simulink model "Detailed_Simulation_recogface_finger_yolo"  (R2023b)
settings: Solver=VariableStepAuto  StartTime=0.0  StopTime=100000  RelTol=1e-3
StartFcn:
  | %url_dc = 'http://localhost:51310/aas/joint_mechanism_1_aas/submodels/joint_mechanism_specific_submodel/elements/DampingCoefficient';
  | %response = webread(url_dc);
  | %set_param('Detailed_Simulation_v15_aas_if_V192_168_179_2/Revolute Joint1/','DampingCoefficient', response.elem.value);
  | %url_lal = 'http://localhost:51310/aas/joint_mechanism_1_aas/submodels/joint_mechanism_specific_submodel/elements/LowerAngleLimit';
  | %response = webread(url_lal);
  | 
  | %set_param('Detailed_Simulation_v15_aas_if_V192_168_179_2/Revolute Joint1/','LowerLimitBound','-45');
undefined symbols (not defined in the file): f, X, Y, Z
libraries: sm_lib x22, nesl_utility x7, slrealtimeutilitieslib x3, instrumentlib x2, slrealtimeiplib x1, dspnetwork x1
settings Model: Creator=Billiet  LastModifiedBy=Zimmermann
settings SolverCC: AutoInsertRateTranBlk=on
settings DebuggingCC: DebugExecutionForFMUViaOutOfProcess=on
settings ModelReferenceCC: EnableRefExpFcnMdlSchedulingChecks=on
settings ExplorerConfigSet: SimMechanicsOpenEditorOnUpdate=off

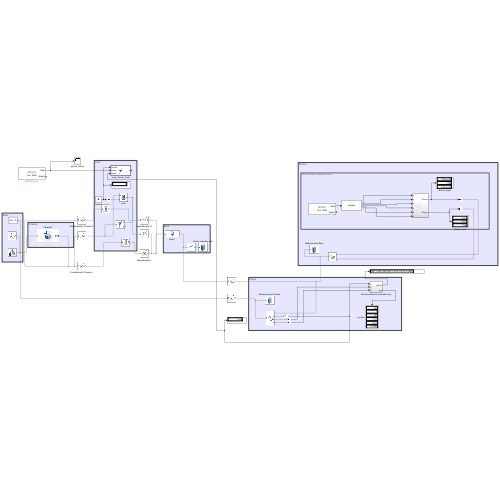
[thumbnail: Simulink's stored preview of the top-level diagram]
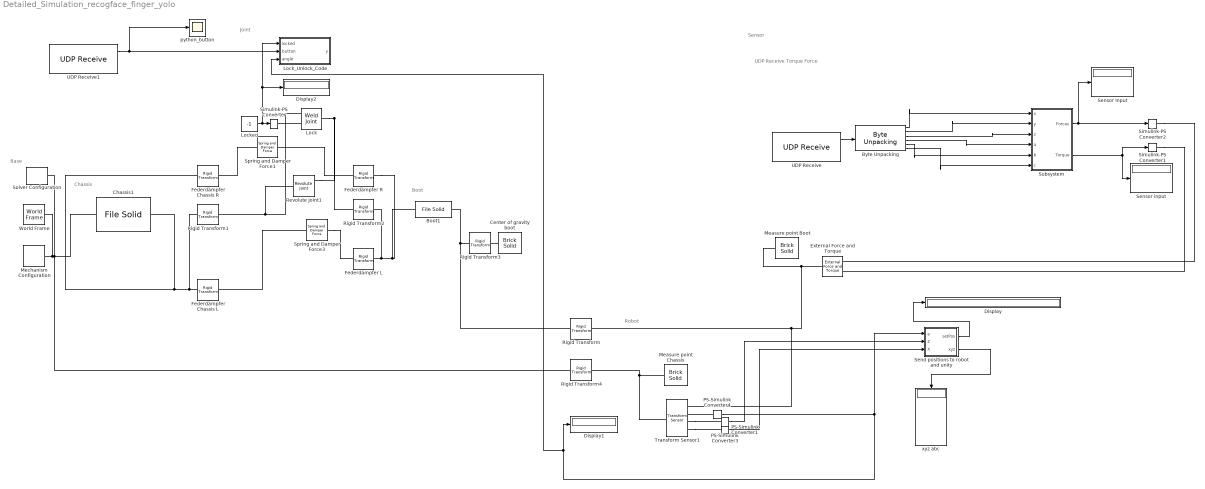
== system Detailed_Simulation_recogface_finger_yolo ==
  note: UDP Receive Torque Force
  note: Robot
  note: Sensor
  note: Base
  note: Boot
  note: Joint
  note: Chassis
  Boot1 : sm_lib/Body Elements/File Solid  ExtGeomFileName=C:\Users\Zimmermann\Desktop\ROBVAR 2.0\04 Simulink\Detailed\3D-Parts\prt\Boot.stl  UnitType=Custom  ExtGeomFileUnits=mm  StepReaderType=HEX  ExportConvexHullGeometry=off  InertiaType=CalculateFromGeometry  Mass=25  MassUnits=kg  CenterOfMass=[0 0 0]  CenterOfMassUnits=m  MomentsOfInertia=[1 1 1]  MomentsOfInertiaUnits=kg*m^2  ProductsOfInertia=[0 0 0]  ProductsOfInertiaUnits=kg*m^2  BasedOnType=Mass  Density=2.7  DensityUnits=g/cm^3  DoExposeReferenceFrame=on  SerializedFrames=<Frames><Frame><Id>Frame1</Id><Value><Name>J</Name><Origin><Source>ReferenceFrame</Source><FeatureName></FeatureName></Origin><PrimaryAxis><DefinedDirection>+Y</DefinedDirection><Source>ReferenceFrame</Source><SourceDirection>+Y</SourceDirection><FeatureName></FeatureName></PrimaryAxis><SecondaryAxis><DefinedDirection>+X</DefinedDirection><Source>ReferenceFrame</Source><SourceDirection>+Z</SourceDirection><FeatureName></FeatureName></SecondaryAxis></Value></Frame></Frames>  GraphicType=FromGeometry  MarkerShape=Sphere  MarkerSize=10  GraphicVisPropType=SimpleVisualProperties  GraphicDiffuseColor=[0.4 0.4 1.0]  GraphicSpecularColor=[0.5 0.5 0.5 1.0]  GraphicAmbientColor=[0.15 0.15 0.15 1.0]  GraphicEmissiveColor=[0.0 0.0 0.0 1.0]  GraphicShininess=75  GraphicOpacity=1.0
  Byte Unpacking : slrealtimeutilitieslib/Byte Unpacking  MaskUnpackedDataTypes={['int32'], ['int32'], ['int32'], ['int32'], ['int32'], ['int32']}  MaskUnpackedDataSizes={[1],[1],[1],[1],[1],[1]}  MaskAlignment=4
  Center of gravity boot : sm_lib/Body Elements/Brick Solid  GraphicAmbientColor=[0.15 0.15 0.15 1.0]  BasedOnType=Density  BrickDimensions=[1 1 1]  BrickDimensionsUnits=mm  CenterOfMass=[0 0 0]  CenterOfMassUnits=m  GraphicDiffuseColor=[0.0 0.0 1.0]  Density=1000  DensityUnits=kg/m^3  DoExposeReferenceFrame=on  GraphicEmissiveColor=[0.0 0.0 0.0 1.0]  ExportEntireGeometry=off  SerializedFrames=<Frames/>  MarkerShape=Sphere  MarkerSize=10  GraphicType=FromGeometry  InertiaType=CalculateFromGeometry  Mass=1  MassUnits=kg  MomentsOfInertia=[1 1 1]  MomentsOfInertiaUnits=kg*m^2  GraphicOpacity=1.0  ProductsOfInertia=[0 0 0]  ProductsOfInertiaUnits=kg*m^2  GraphicShininess=75  GraphicSpecularColor=[0.5 0.5 0.5 1.0]  GraphicVisPropType=SimpleVisualProperties
  Chassis1 : sm_lib/Body Elements/File Solid  ExtGeomFileName=C:\Users\Zimmermann\Desktop\ROBVAR 2.0\04 Simulink\Detailed\3D-Parts\prt\Chassis.stl  UnitType=Custom  ExtGeomFileUnits=mm  StepReaderType=HEX  ExportConvexHullGeometry=off  InertiaType=CalculateFromGeometry  Mass=600  MassUnits=kg  CenterOfMass=[0 0 0]  CenterOfMassUnits=m  MomentsOfInertia=[1 1 1]  MomentsOfInertiaUnits=kg*m^2  ProductsOfInertia=[0 0 0]  ProductsOfInertiaUnits=kg*m^2  BasedOnType=Density  Density=2.7  DensityUnits=g/cm^3  DoExposeReferenceFrame=on  SerializedFrames=<Frames><Frame><Id>Frame1</Id><Value><Name>joint</Name><Origin><Source>ReferenceFrame</Source><FeatureName></FeatureName></Origin><PrimaryAxis><DefinedDirection>+Y</DefinedDirection><Source>ReferenceFrame</Source><SourceDirection>+Y</SourceDirection><FeatureName></FeatureName></PrimaryAxis><SecondaryAxis><DefinedDirection>-X</DefinedDirection><Source>ReferenceFrame</Source><SourceDirection>-Z</SourceDirection><FeatureName></FeatureName></SecondaryAxis></Value></Frame></Frames>  GraphicType=FromGeometry  MarkerShape=Sphere  MarkerSize=10  GraphicVisPropType=SimpleVisualProperties  GraphicDiffuseColor=[1.0 0.6 0.0]  GraphicSpecularColor=[0.5 0.5 0.5 1.0]  GraphicAmbientColor=[0.15 0.15 0.15 1.0]  GraphicEmissiveColor=[0.0 0.0 0.0 1.0]  GraphicShininess=75  GraphicOpacity=1.0
  Display : Display
  Display1 : Display
  Display2 : Display
  External Force and Torque : sm_lib/Forces and Torques/External Force and Torque  ForceResolutionFrame=AttachedFrame  EnableForceX=off  EnableForceY=off  EnableForceZ=off  EnableForce=on  TorqueResolutionFrame=AttachedFrame  EnableTorqueX=off  EnableTorqueY=off  EnableTorqueZ=off  EnableTorque=on
  Federdämpfer Chassis L : sm_lib/Frames and Transforms/Rigid Transform  TranslationMethod=Cartesian  TranslationStandardOffset=0  TranslationStandardOffsetUnits=mm  TranslationStandardAxis=+Z  TranslationCartesianOffset=[-2055 0 -660]  TranslationCartesianOffsetUnits=mm  TranslationROffset=0  TranslationROffsetUnits=m  TranslationZOffset=0  TranslationZOffsetUnits=m  TranslationThetaOffset=0  TranslationThetaOffsetUnits=deg  RotationMethod=None  RotationAngleUnits=deg  RotationStandardAxis=+Z  RotationAngle=0.0  RotationArbitraryAxis=[0 0 1]  FollAlignAxisA=+X  BaseAlignAxisA=+Y  FollAlignAxisB=+Y  BaseAlignAxisB=+Z  RotationSequenceAxes=FollowerAxes  RotationSequence=XYX  RotationSequenceAngles=[0 0 0]  RotationSequenceAnglesUnits=deg  RotationMatrix=[1 0 0; 0 1 0; 0 0 1]  Quaternion=[1 0 0 0]
  Federdämpfer Chassis R : sm_lib/Frames and Transforms/Rigid Transform  TranslationMethod=Cartesian  TranslationStandardOffset=0  TranslationStandardOffsetUnits=mm  TranslationStandardAxis=+Z  TranslationCartesianOffset=[-2055 70 660]  TranslationCartesianOffsetUnits=mm  TranslationROffset=0  TranslationROffsetUnits=m  TranslationZOffset=0  TranslationZOffsetUnits=m  TranslationThetaOffset=0  TranslationThetaOffsetUnits=deg  RotationMethod=None  RotationAngleUnits=deg  RotationStandardAxis=+Z  RotationAngle=0.0  RotationArbitraryAxis=[0 0 1]  FollAlignAxisA=+X  BaseAlignAxisA=+Y  FollAlignAxisB=+Y  BaseAlignAxisB=+Z  RotationSequenceAxes=FollowerAxes  RotationSequence=XYX  RotationSequenceAngles=[0 0 0]  RotationSequenceAnglesUnits=deg  RotationMatrix=[1 0 0; 0 1 0; 0 0 1]  Quaternion=[1 0 0 0]
  Federdämpfer L : sm_lib/Frames and Transforms/Rigid Transform  TranslationMethod=Cartesian  TranslationStandardOffset=0  TranslationStandardOffsetUnits=mm  TranslationStandardAxis=+Z  TranslationCartesianOffset=[1829 -280 660]  TranslationCartesianOffsetUnits=mm  TranslationROffset=0  TranslationROffsetUnits=m  TranslationZOffset=0  TranslationZOffsetUnits=m  TranslationThetaOffset=0  TranslationThetaOffsetUnits=deg  RotationMethod=None  RotationAngleUnits=deg  RotationStandardAxis=+Z  RotationAngle=0.0  RotationArbitraryAxis=[0 0 1]  FollAlignAxisA=+X  BaseAlignAxisA=+Y  FollAlignAxisB=+Y  BaseAlignAxisB=+Z  RotationSequenceAxes=FollowerAxes  RotationSequence=XYX  RotationSequenceAngles=[0 0 0]  RotationSequenceAnglesUnits=deg  RotationMatrix=[1 0 0; 0 1 0; 0 0 1]  Quaternion=[1 0 0 0]
  Federdämpfer R : sm_lib/Frames and Transforms/Rigid Transform  TranslationMethod=Cartesian  TranslationStandardOffset=0  TranslationStandardOffsetUnits=mm  TranslationStandardAxis=+Z  TranslationCartesianOffset=[1829 -280 -660]  TranslationCartesianOffsetUnits=mm  TranslationROffset=0  TranslationROffsetUnits=m  TranslationZOffset=0  TranslationZOffsetUnits=m  TranslationThetaOffset=0  TranslationThetaOffsetUnits=deg  RotationMethod=None  RotationAngleUnits=deg  RotationStandardAxis=+Z  RotationAngle=0.0  RotationArbitraryAxis=[0 0 1]  FollAlignAxisA=+X  BaseAlignAxisA=+Y  FollAlignAxisB=+Y  BaseAlignAxisB=+Z  RotationSequenceAxes=FollowerAxes  RotationSequence=XYX  RotationSequenceAngles=[0 0 0]  RotationSequenceAnglesUnits=deg  RotationMatrix=[1 0 0; 0 1 0; 0 0 1]  Quaternion=[1 0 0 0]
  Lock : sm_lib/Joints/Weld Joint  JointMode=ProvidedByInput  SenseConstraintForce=off  SenseConstraintForceX=off  SenseConstraintForceY=off  SenseConstraintForceZ=off  SenseConstraintTorque=off  SenseConstraintTorqueX=off  SenseConstraintTorqueY=off  SenseConstraintTorqueZ=off  SenseTotalForce=off  SenseTotalForceX=off  SenseTotalForceY=off  SenseTotalForceZ=off  SenseTotalTorque=off  SenseTotalTorqueX=off  SenseTotalTorqueY=off  SenseTotalTorqueZ=off  CompositeWrenchDir=FollowerOnBase  CompositeWrenchFrame=BaseFrame
  Lock_Unlock_Code : MATLAB Function  TreatAsAtomicUnit=on
  Locked : Constant  Value=-1
  Measure point Boot : sm_lib/Body Elements/Brick Solid  GraphicAmbientColor=[0.15 0.15 0.15 1.0]  BasedOnType=Density  BrickDimensions=[1 1 0.1]  BrickDimensionsUnits=cm  CenterOfMass=[0 0 0]  CenterOfMassUnits=m  GraphicDiffuseColor=[1.0 0.0 1.0]  Density=1000  DensityUnits=kg/m^3  DoExposeReferenceFrame=on  GraphicEmissiveColor=[0.0 0.0 0.0 1.0]  ExportEntireGeometry=off  SerializedFrames=<Frames/>  MarkerShape=Sphere  MarkerSize=10  GraphicType=FromGeometry  InertiaType=CalculateFromGeometry  Mass=1  MassUnits=kg  MomentsOfInertia=[1 1 1]  MomentsOfInertiaUnits=kg*m^2  GraphicOpacity=1.0  ProductsOfInertia=[0 0 0]  ProductsOfInertiaUnits=kg*m^2  GraphicShininess=75  GraphicSpecularColor=[0.5 0.5 0.5 1.0]  GraphicVisPropType=SimpleVisualProperties
  Measure point Chassis : sm_lib/Body Elements/Brick Solid  GraphicAmbientColor=[0.15 0.15 0.15 1.0]  BasedOnType=Density  BrickDimensions=[1 1 0.1]  BrickDimensionsUnits=cm  CenterOfMass=[0 0 0]  CenterOfMassUnits=m  GraphicDiffuseColor=[1.0 0.0 1.0]  Density=1000  DensityUnits=kg/m^3  DoExposeReferenceFrame=on  GraphicEmissiveColor=[0.0 0.0 0.0 1.0]  ExportEntireGeometry=off  SerializedFrames=<Frames/>  MarkerShape=Sphere  MarkerSize=10  GraphicType=FromGeometry  InertiaType=CalculateFromGeometry  Mass=1  MassUnits=kg  MomentsOfInertia=[1 1 1]  MomentsOfInertiaUnits=kg*m^2  GraphicOpacity=1.0  ProductsOfInertia=[0 0 0]  ProductsOfInertiaUnits=kg*m^2  GraphicShininess=75  GraphicSpecularColor=[0.5 0.5 0.5 1.0]  GraphicVisPropType=SimpleVisualProperties
  Mechanism Configuration : sm_lib/Utilities/Mechanism Configuration  UniformGravity=Constant  GravityVector=[0 -9.80665 0]  GravityVectorUnits=m/s^2  LinearizationDelta=0.001  JointModeTransitionNonlinearIterations=2
  PS-Simulink Converter1 : nesl_utility/PS-Simulink Converter  PhysicalDomain=network_engine_domain  SubClassName=ps_output  LeftPortType=input  RightPortType=output  PseudoPeriodic=off  Frequencies=[]  VectorFormat=inherit  Unit=inherit  AffineConversion=off
  PS-Simulink Converter3 : nesl_utility/PS-Simulink Converter  PhysicalDomain=network_engine_domain  SubClassName=ps_output  LeftPortType=input  RightPortType=output  PseudoPeriodic=off  Frequencies=[]  VectorFormat=inherit  Unit=inherit  AffineConversion=off
  PS-Simulink Converter4 : nesl_utility/PS-Simulink Converter  PhysicalDomain=network_engine_domain  SubClassName=ps_output  LeftPortType=input  RightPortType=output  PseudoPeriodic=off  Frequencies=[]  VectorFormat=inherit  Unit=inherit  AffineConversion=off
  Revolute Joint1 : sm_lib/Joints/Revolute Joint  JointMode=Normal  SenseConstraintForce=off  SenseConstraintForceX=off  SenseConstraintForceY=off  SenseConstraintForceZ=off  SenseConstraintTorque=off  SenseConstraintTorqueX=off  SenseConstraintTorqueY=off  SenseConstraintTorqueZ=off  SenseTotalForce=off  SenseTotalForceX=off  SenseTotalForceY=off  SenseTotalForceZ=off  SenseTotalTorque=off  SenseTotalTorqueX=off  SenseTotalTorqueY=off  SenseTotalTorqueZ=off  CompositeWrenchDir=FollowerOnBase  CompositeWrenchFrame=BaseFrame  EquilibriumPosition=0  EquilibriumPositionUnits=deg  SpringStiffness=0  SpringStiffnessUnits=N*m/deg  DampingCoefficient=60  DampingCoefficientUnits=N*m/(deg/s)  TorqueActuationMode=NoTorque  MotionActuationMode=ComputedMotion  SensePosition=off  SenseVelocity=on  SenseAcceleration=off  SenseTorqueForce=off  SenseLowerLimitTorqueForce=off  SenseUpperLimitTorqueForce=off  LowerLimitSpecify=on  LowerLimitBound=-75  LowerLimitBoundUnits=deg  LowerLimitStiffness=1e8  LowerLimitStiffnessUnits=N*m/deg  LowerLimitDamping=1000  LowerLimitDampingUnits=N*m/(deg/s)  LowerLimitTransitionRegionWidth=0.1  LowerLimitTransitionRegionWidthUnits=deg  UpperLimitSpecify=on  UpperLimitBound=0  UpperLimitBoundUnits=deg  UpperLimitStiffness=1e8  UpperLimitStiffnessUnits=N*m/deg  UpperLimitDamping=1000  UpperLimitDampingUnits=N*m/(deg/s)  UpperLimitTransitionRegionWidth=0.1  UpperLimitTransitionRegionWidthUnits=deg  PositionTargetSpecify=off  PositionTargetPriority=High  PositionTargetValue=0  PositionTargetValueUnits=deg  VelocityTargetSpecify=off  VelocityTargetPriority=Low  VelocityTargetValue=100  VelocityTargetValueUnits=deg/s
  Rigid Transform : sm_lib/Frames and Transforms/Rigid Transform  TranslationMethod=Cartesian  TranslationStandardOffset=0  TranslationStandardOffsetUnits=mm  TranslationStandardAxis=+Z  TranslationCartesianOffset=[0 298.5 -2150]  TranslationCartesianOffsetUnits=mm  TranslationROffset=0  TranslationROffsetUnits=m  TranslationZOffset=0  TranslationZOffsetUnits=m  TranslationThetaOffset=0  TranslationThetaOffsetUnits=deg  RotationMethod=StandardAxis  RotationAngleUnits=deg  RotationStandardAxis=+X  RotationAngle=90  RotationArbitraryAxis=[0 0 1]  FollAlignAxisA=+X  BaseAlignAxisA=+Y  FollAlignAxisB=+Y  BaseAlignAxisB=+Z  RotationSequenceAxes=FollowerAxes  RotationSequence=XYX  RotationSequenceAngles=[0 0 0]  RotationSequenceAnglesUnits=deg  RotationMatrix=[1 0 0; 0 1 0; 0 0 1]  Quaternion=[1 0 0 0]
  Rigid Transform1 : sm_lib/Frames and Transforms/Rigid Transform  TranslationMethod=Cartesian  TranslationStandardOffset=260  TranslationStandardOffsetUnits=mm  TranslationStandardAxis=+X  TranslationCartesianOffset=[-1680 291.9 725]  TranslationCartesianOffsetUnits=mm  TranslationROffset=0  TranslationROffsetUnits=m  TranslationZOffset=0  TranslationZOffsetUnits=m  TranslationThetaOffset=0  TranslationThetaOffsetUnits=deg  RotationMethod=None  RotationAngleUnits=deg  RotationStandardAxis=+Z  RotationAngle=0.0  RotationArbitraryAxis=[0 0 1]  FollAlignAxisA=+X  BaseAlignAxisA=+Y  FollAlignAxisB=+Y  BaseAlignAxisB=+Z  RotationSequenceAxes=FollowerAxes  RotationSequence=XYX  RotationSequenceAngles=[0 0 0]  RotationSequenceAnglesUnits=deg  RotationMatrix=[1 0 0; 0 1 0; 0 0 1]  Quaternion=[1 0 0 0]
  Rigid Transform2 : sm_lib/Frames and Transforms/Rigid Transform  TranslationMethod=Cartesian  TranslationStandardOffset=260  TranslationStandardOffsetUnits=mm  TranslationStandardAxis=+X  TranslationCartesianOffset=[1675 -296 -725]  TranslationCartesianOffsetUnits=mm  TranslationROffset=0  TranslationROffsetUnits=m  TranslationZOffset=0  TranslationZOffsetUnits=m  TranslationThetaOffset=0  TranslationThetaOffsetUnits=deg  RotationMethod=None  RotationAngleUnits=deg  RotationStandardAxis=+Y  RotationAngle=-90  RotationArbitraryAxis=[0 0 1]  FollAlignAxisA=+X  BaseAlignAxisA=-Z  FollAlignAxisB=+Y  BaseAlignAxisB=+Z  RotationSequenceAxes=FollowerAxes  RotationSequence=XYX  RotationSequenceAngles=[0 0 0]  RotationSequenceAnglesUnits=deg  RotationMatrix=[1 0 0; 0 1 0; 0 0 1]  Quaternion=[1 0 0 0]
  Rigid Transform3 : sm_lib/Frames and Transforms/Rigid Transform  TranslationMethod=Cartesian  TranslationStandardOffset=0  TranslationStandardOffsetUnits=mm  TranslationStandardAxis=+Z  TranslationCartesianOffset=[0 140 -2150]  TranslationCartesianOffsetUnits=mm  TranslationROffset=0  TranslationROffsetUnits=m  TranslationZOffset=0  TranslationZOffsetUnits=m  TranslationThetaOffset=0  TranslationThetaOffsetUnits=deg  RotationMethod=RotationSequence  RotationAngleUnits=deg  RotationStandardAxis=+X  RotationAngle=90  RotationArbitraryAxis=[0 0 1]  FollAlignAxisA=+X  BaseAlignAxisA=+Y  FollAlignAxisB=+Y  BaseAlignAxisB=+Z  RotationSequenceAxes=FollowerAxes  RotationSequence=YZX  RotationSequenceAngles=[90 0 0]  RotationSequenceAnglesUnits=deg  RotationMatrix=[1 0 0; 0 1 0; 0 0 1]  Quaternion=[1 0 0 0]
  Rigid Transform4 : sm_lib/Frames and Transforms/Rigid Transform  TranslationMethod=Cartesian  TranslationStandardOffset=0  TranslationStandardOffsetUnits=mm  TranslationStandardAxis=+Z  TranslationCartesianOffset=[0 294.4 -2155]  TranslationCartesianOffsetUnits=mm  TranslationROffset=0  TranslationROffsetUnits=m  TranslationZOffset=0  TranslationZOffsetUnits=m  TranslationThetaOffset=0  TranslationThetaOffsetUnits=deg  RotationMethod=StandardAxis  RotationAngleUnits=deg  RotationStandardAxis=+X  RotationAngle=90  RotationArbitraryAxis=[0 0 1]  FollAlignAxisA=+X  BaseAlignAxisA=+Y  FollAlignAxisB=+Y  BaseAlignAxisB=+Z  RotationSequenceAxes=FollowerAxes  RotationSequence=XYX  RotationSequenceAngles=[0 0 0]  RotationSequenceAnglesUnits=deg  RotationMatrix=[1 0 0; 0 1 0; 0 0 1]  Quaternion=[1 0 0 0]
  Send positions to robot and unity : Subsystem
  Sensor Input : Display
  Sensor input : Display
  Simulink-PS Converter : nesl_utility/Simulink-PS Converter  PhysicalDomain=network_engine_domain  SubClassName=ps_input  LeftPortType=input  RightPortType=output  PseudoPeriodic=off  Frequencies=[]  NoiseDistribution=none  NoiseParameters=[]  Unit=1  AffineConversion=off  FilteringAndDerivatives=provide  SimscapeFilterOrder=1  InputFilterTimeConstant=0.001  UdotUserProvided=0
  Simulink-PS Converter1 : nesl_utility/Simulink-PS Converter  PhysicalDomain=network_engine_domain  SubClassName=ps_input  LeftPortType=input  RightPortType=output  PseudoPeriodic=off  Frequencies=[]  NoiseDistribution=none  NoiseParameters=[]  Unit=1  AffineConversion=off  FilteringAndDerivatives=provide  SimscapeFilterOrder=1  InputFilterTimeConstant=0.001  UdotUserProvided=0
  Simulink-PS Converter2 : nesl_utility/Simulink-PS Converter  PhysicalDomain=network_engine_domain  SubClassName=ps_input  LeftPortType=input  RightPortType=output  PseudoPeriodic=off  Frequencies=[]  NoiseDistribution=none  NoiseParameters=[]  Unit=1  AffineConversion=off  FilteringAndDerivatives=provide  SimscapeFilterOrder=1  InputFilterTimeConstant=0.001  UdotUserProvided=0
  Solver Configuration : nesl_utility/Solver Configuration  PhysicalDomain=network_engine_domain  SubClassName=solver  LeftPortType=input  RightPortType=generic  Tones=[]  Harmonics=[]  SimulateNoise=off  Profile=off  UseLocalSampling=off  EnableSwitchedLinearOptims=on  FrequencyDomain=off  UseCCode=off  RelTol=0.001  AbsTol=1e-06  MinStep=1e-09  ToWorkspace=off  RevertToSquareIcSolve=off  NumHomotopyIterations=100  PhasorMode=off  PhasorModeNumHarmonics=1  ConsistencySolver=NEWTON_FTOL  IndexReductionMethod=DerivativeReplacement  DoDC=off  ResidualTolerance=1e-09  ConsistencyTolSource=GLOBAL  ConsistencyAbsTol=0.001  ConsistencyRelTol=0.001  ConsistencyTolFactor=0.001  UseLocalSolver=off  LocalSolverChoice=NE_BACKWARD_EULER_ADVANCER  ResolveIndetEquations=on  FunctionEvalNumThread=1  LocalSolverSampleTime=0.001  DoFixedCost=off  MaxNonlinIter=3  MaxModeIter=2  ComputeImpulses=off  ImpulseIterations=2  LinearAlgebra=Sparse  LinearAlgebraNumThread=0  EquationFormulation=NE_TIME_EF  DelaysMemoryBudget=1024  AutomaticFiltering=on  FilteringTimeConstant=0.001  PartitionStorageMethod=AS_NEEDED  PartitionMemoryBudget=1024  PartitionMethod=FAST  MultibodyUseLocalSolver=off  MultibodyLocalSolverChoice=ODE1  MultibodyLocalSolverSampleTime=0.001
  Spring and Damper Force1 : sm_lib/Forces and Torques/Spring and Damper Force  NaturalLength=9  NaturalLengthUnits=m  SpringStiffness=6000  SpringStiffnessUnits=N/m  DampingCoefficient=600000  DampingCoefficientUnits=N/(m/s)  SenseForce=off
  Spring and Damper Force3 : sm_lib/Forces and Torques/Spring and Damper Force  NaturalLength=9  NaturalLengthUnits=m  SpringStiffness=6000  SpringStiffnessUnits=N/m  DampingCoefficient=600000  DampingCoefficientUnits=N/(m/s)  SenseForce=off
  Subsystem : Subsystem
  Transform Sensor1 : sm_lib/Frames and Transforms/Transform Sensor  MeasurementFrame=World  RotationSequence=XYX  SenseAngle=on  SenseAxis=off  SenseQ=off  SenseR=off  SenseRotationSequence=off  SenseOmegaX=off  SenseOmegaY=off  SenseOmegaZ=off  SenseOmega=off  SenseQDot=off  SenseRDot=off  SenseRotationSequenceDot=off  SenseAlphaX=off  SenseAlphaY=off  SenseAlphaZ=off  SenseAlpha=off  SenseQDDot=off  SenseRDDot=off  SenseX=off  SenseY=on  SenseZ=on  SenseXYZ=off  SenseRad=off  SenseAzim=off  SenseDist=off  SenseInc=off  SenseXDot=off  SenseYDot=off  SenseZDot=off  SenseXYZDot=off  SenseRadDot=off  SenseAzimDot=off  SenseDistDot=off  SenseIncDot=off  SenseXDDot=off  SenseYDDot=off  SenseZDDot=off  SenseXYZDDot=off  SenseRadDDot=off  SenseAzimDDot=off  SenseDistDDot=off  SenseIncDDot=off
  UDP Receive : instrumentlib/UDP Receive  LocalAddress=127.0.0.1  LocalPort=7890  EnablePortSharing=off  Host=localhost  Port=7890  GetLatestData=on  DataSize="[1  24]"  DataType=uint8  ASCIIFormatting=%f,  Terminator=LF  CustomTerminator=10  ByteOrder=big-endian  EnableBlockingMode=off  Timeout=10  SampleTime=0.04  SimulateUsing=Interpreted execution
  UDP Receive1 : instrumentlib/UDP Receive  LocalAddress=127.0.0.1  LocalPort=5005  EnablePortSharing=off  Host=localhost  Port=9090  GetLatestData=on  DataSize=[1]  DataType=uint8  ASCIIFormatting=%f,  Terminator=LF  CustomTerminator=10  ByteOrder=big-endian  EnableBlockingMode=off  Timeout=10  SampleTime=0.05  SimulateUsing=Interpreted execution
  World Frame : sm_lib/Frames and Transforms/World Frame
  python_button : Scope
  xyz abc : Display
  wires:
  PS-Simulink Converter4/1 -> Send positions to robot and unity/1(a), Lock_Unlock_Code/3(angle), Display1/1
  Send positions to robot and unity/2(xyz) -> xyz abc/1
  Send positions to robot and unity/1(setPos) -> Display/1
  Locked/1 -> Lock_Unlock_Code/1(locked), Display2/1, Simulink-PS Converter/1
  PS-Simulink Converter1/1 -> Send positions to robot and unity/3(X)
  PS-Simulink Converter3/1 -> Send positions to robot and unity/2(Z)
  Subsystem/2(Torque) -> Simulink-PS Converter1/1, Sensor input/1
  Subsystem/1(Forces) -> Sensor Input/1, Simulink-PS Converter2/1
  UDP Receive/1 -> Byte Unpacking/1
  Byte Unpacking/3 -> Subsystem/3(z)
  Byte Unpacking/2 -> Subsystem/2(y)
  Byte Unpacking/1 -> Subsystem/1(x)
  Byte Unpacking/6 -> Subsystem/6(c)
  Byte Unpacking/5 -> Subsystem/5(b)
  Byte Unpacking/4 -> Subsystem/4(a)
  UDP Receive1/1 -> Lock_Unlock_Code/2(button), python_button/1
  connections:
  Chassis1/RConn1 -- Mechanism Configuration/RConn1 -- World Frame/RConn1 -- Rigid Transform4/LConn1 -- Solver Configuration/RConn1
  PS-Simulink Converter4/LConn1 -- Transform Sensor1/RConn2
  Transform Sensor1/RConn3 -- PS-Simulink Converter3/LConn1
  Transform Sensor1/RConn4 -- PS-Simulink Converter1/LConn1
  Simulink-PS Converter1/RConn1 -- External Force and Torque/LConn2
  Simulink-PS Converter2/RConn1 -- External Force and Torque/LConn1
  Lock/LConn2 -- Simulink-PS Converter/RConn1
  Spring and Damper Force3/RConn1 -- Federdämpfer L/LConn1
  Spring and Damper Force1/RConn1 -- Federdämpfer R/LConn1
  Revolute Joint1/RConn1 -- Lock/RConn1 -- Rigid Transform2/LConn1
  Rigid Transform2/RConn1 -- Federdämpfer R/RConn1 -- Boot1/LConn1 -- Federdämpfer L/RConn1
  Center of gravity boot/RConn1 -- Rigid Transform3/RConn1
  Measure point Boot/RConn1 -- External Force and Torque/RConn1 -- Transform Sensor1/RConn1 -- Rigid Transform/RConn1
  Rigid Transform/LConn1 -- Boot1/RConn1 -- Rigid Transform3/LConn1
  Spring and Damper Force3/LConn1 -- Federdämpfer Chassis L/RConn1
  Spring and Damper Force1/LConn1 -- Federdämpfer Chassis R/RConn1
  Lock/LConn1 -- Rigid Transform1/RConn1 -- Revolute Joint1/LConn1
  Rigid Transform1/LConn1 -- Federdämpfer Chassis R/LConn1 -- Chassis1/LConn1 -- Federdämpfer Chassis L/LConn1
  Measure point Chassis/RConn1 -- Rigid Transform4/RConn1 -- Transform Sensor1/LConn1

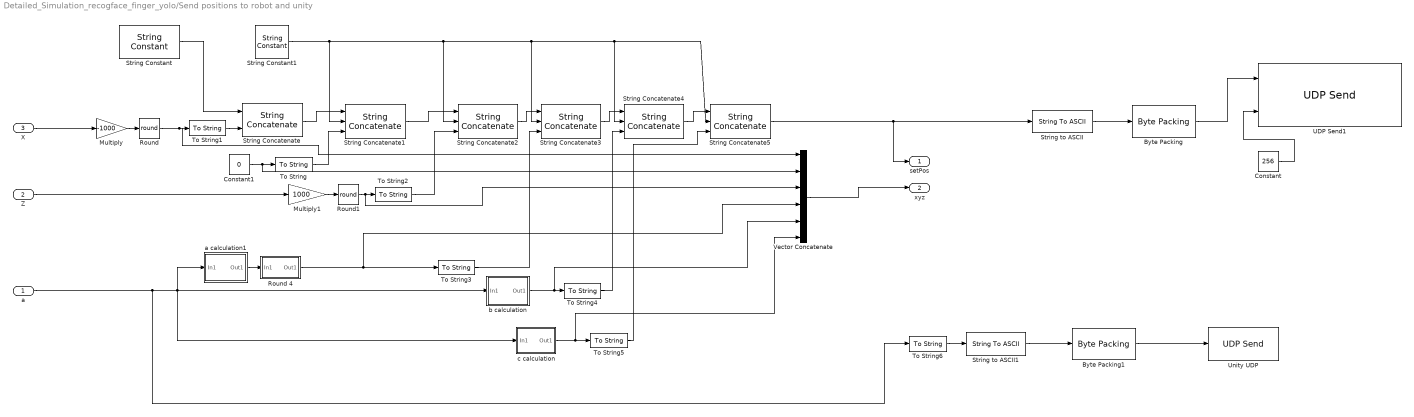
== system Detailed_Simulation_recogface_finger_yolo/Send positions to robot and unity ==
  a : Inport
  Z : Inport  Port=2
  X : Inport  Port=3
  Byte Packing : slrealtimeutilitieslib/Byte Packing  MaskPackedDataType=uint8  MaskUnpackedDataTypes={'uint8'}  MaskAlignment=1
  Byte Packing1 : slrealtimeutilitieslib/Byte Packing  MaskPackedDataType=uint8  MaskUnpackedDataTypes={'uint8'}  MaskAlignment=1
  Constant : Constant  Value=256
  Constant1 : Constant  Value=0
  Multiply : Gain  Gain=-1000
  Multiply1 : Gain  Gain=1000
  Round : Rounding  Operator=round
  Round 4 : Subsystem
  Round1 : Rounding  Operator=round
  String Concatenate : StringConcatenate
  String Concatenate{1..5} (5 alike) : StringConcatenate  Inputs=3
  String Constant : StringConstant  String="\"SET_POS,\""
  String Constant1 : StringConstant  String="\",\""
  String to ASCII : StringToASCII  OutputVectorSize=64
  String to ASCII1 : StringToASCII  OutputVectorSize=64
  To String{,1..6} (7 alike) : ToString
  UDP Send1 : slrealtimeiplib/UDP Send  useHostTargetConn=off  toAddress='127.0.0.1'  toPort=5554  sampleTime=-1  enableMessage=off
  Unity UDP : dspnetwork/UDP Send  remoteURL='127.0.0.1'  remotePort=8889  localURL='0.0.0.0'  localPortSource=Automatically determine  localPort=-1  sendBufferSize=512  sampletime=-1  blockPlatform=[]  separateLengthPort=0
  Vector Concatenate : Concatenate  NumInputs=6
  a calculation1 : Subsystem
  b calculation : Subsystem
  c calculation : Subsystem
  setPos : Outport
  xyz : Outport  Port=2
  wires:
  String Constant1/1 -> String Concatenate5/2, String Concatenate4/2, String Concatenate3/2, String Concatenate2/2, String Concatenate1/2
  String Concatenate4/1 -> String Concatenate5/1
  Constant1/1 -> Vector Concatenate/2, To String/1
  String Constant/1 -> String Concatenate/1
  String Concatenate1/1 -> String Concatenate2/1
  String Concatenate3/1 -> String Concatenate4/1
  String Concatenate2/1 -> String Concatenate3/1
  String Concatenate/1 -> String Concatenate1/1
  To String/1 -> String Concatenate1/3
  X/1 -> Multiply/1
  Z/1 -> Multiply1/1
  To String1/1 -> String Concatenate/2
  To String2/1 -> String Concatenate2/3
  Multiply/1 -> Round/1
  To String3/1 -> String Concatenate3/3
  a/1 -> To String6/1, c calculation/1(In1), b calculation/1(In1), a calculation1/1(In1)
  To String4/1 -> String Concatenate4/3
  To String5/1 -> String Concatenate5/3
  b calculation/1(Out1) -> Vector Concatenate/5, To String4/1
  c calculation/1(Out1) -> Vector Concatenate/6, To String5/1
  Vector Concatenate/1 -> xyz/1
  Multiply1/1 -> Round1/1
  Round/1 -> Vector Concatenate/1, To String1/1
  Round1/1 -> Vector Concatenate/3, To String2/1
  Round 4/1(Out1) -> Vector Concatenate/4, To String3/1
  a calculation1/1(Out1) -> Round 4/1(In1)
  To String6/1 -> String to ASCII1/1
  String to ASCII1/1 -> Byte Packing1/1
  Byte Packing1/1 -> Unity UDP/1
  String to ASCII/1 -> Byte Packing/1
  String Concatenate5/1 -> String to ASCII/1, setPos/1
  Byte Packing/1 -> UDP Send1/1
  Constant/1 -> UDP Send1/2

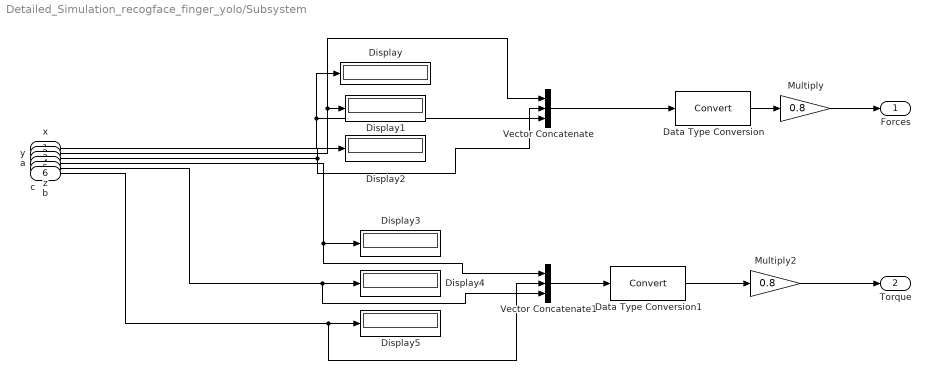
== system Detailed_Simulation_recogface_finger_yolo/Subsystem ==
  x : Inport
  y : Inport  Port=2
  z : Inport  Port=3
  a : Inport  Port=4
  b : Inport  Port=5
  c : Inport  Port=6
  Data Type Conversion : DataTypeConversion  SaturateOnIntegerOverflow=off  RndMeth=Floor
  Data Type Conversion1 : DataTypeConversion  SaturateOnIntegerOverflow=off  RndMeth=Floor
  Display{,1..5} (6 alike) : Display
  Multiply : Gain  Gain=0.8
  Multiply2 : Gain  Gain=0.8
  Vector Concatenate : Concatenate  NumInputs=3
  Vector Concatenate1 : Concatenate  NumInputs=3
  Forces : Outport
  Torque : Outport  Port=2
  wires:
  b/1 -> Vector Concatenate1/3, Display4/1
  Data Type Conversion/1 -> Multiply/1
  y/1 -> Vector Concatenate/1, Display1/1
  c/1 -> Vector Concatenate1/2, Display5/1
  Data Type Conversion1/1 -> Multiply2/1
  Vector Concatenate1/1 -> Data Type Conversion1/1
  a/1 -> Vector Concatenate1/1, Display3/1
  x/1 -> Display/1, Vector Concatenate/3
  Multiply2/1 -> Torque/1
  Vector Concatenate/1 -> Data Type Conversion/1
  z/1 -> Display2/1, Vector Concatenate/2
  Multiply/1 -> Forces/1

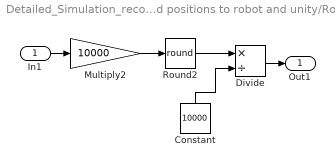
== system Detailed_Simulation_recogface_finger_yolo/Send positions to robot and unity/Round 4 ==
  In1 : Inport
  Constant : Constant  Value=10000
  Divide : Product  Inputs=*/
  Multiply2 : Gain  Gain=10000
  Round2 : Rounding  Operator=round
  Out1 : Outport
  wires:
  Round2/1 -> Divide/1
  Constant/1 -> Divide/2
  Multiply2/1 -> Round2/1
  Divide/1 -> Out1/1
  In1/1 -> Multiply2/1

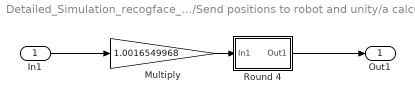
== system Detailed_Simulation_recogface_finger_yolo/Send positions to robot and unity/a calculation1 ==
  In1 : Inport
  Multiply : Gain  Gain=1.0016549968
  Round 4 : Subsystem
  Out1 : Outport
  wires:
  Round 4/1(Out1) -> Out1/1
  In1/1 -> Multiply/1
  Multiply/1 -> Round 4/1(In1)

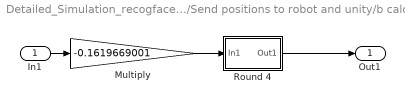
== system Detailed_Simulation_recogface_finger_yolo/Send positions to robot and unity/b calculation ==
  In1 : Inport
  Multiply : Gain  Gain=-0.1619669001
  Round 4 : Subsystem
  Out1 : Outport
  wires:
  Round 4/1(Out1) -> Out1/1
  In1/1 -> Multiply/1
  Multiply/1 -> Round 4/1(In1)

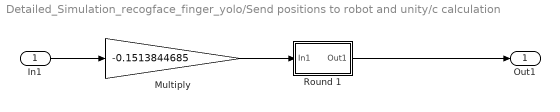
== system Detailed_Simulation_recogface_finger_yolo/Send positions to robot and unity/c calculation ==
  In1 : Inport
  Multiply : Gain  Gain=-0.1513844685
  Round 1 : Subsystem
  Out1 : Outport
  wires:
  Round 1/1(Out1) -> Out1/1
  In1/1 -> Multiply/1
  Multiply/1 -> Round 1/1(In1)

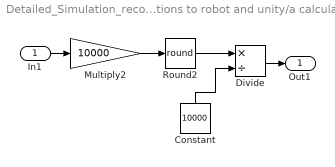
== system Detailed_Simulation_recogface_finger_yolo/Send positions to robot and unity/a calculation1/Round 4 ==
  In1 : Inport
  Constant : Constant  Value=10000
  Divide : Product  Inputs=*/
  Multiply2 : Gain  Gain=10000
  Round2 : Rounding  Operator=round
  Out1 : Outport
  wires:
  Round2/1 -> Divide/1
  Constant/1 -> Divide/2
  Multiply2/1 -> Round2/1
  Divide/1 -> Out1/1
  In1/1 -> Multiply2/1

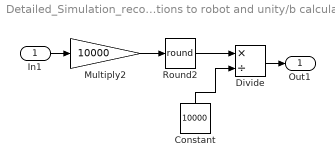
== system Detailed_Simulation_recogface_finger_yolo/Send positions to robot and unity/b calculation/Round 4 ==
  In1 : Inport
  Constant : Constant  Value=10000
  Divide : Product  Inputs=*/
  Multiply2 : Gain  Gain=10000
  Round2 : Rounding  Operator=round
  Out1 : Outport
  wires:
  Round2/1 -> Divide/1
  Constant/1 -> Divide/2
  Multiply2/1 -> Round2/1
  Divide/1 -> Out1/1
  In1/1 -> Multiply2/1

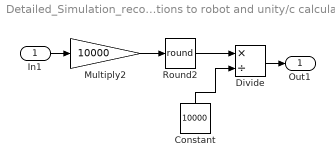
== system Detailed_Simulation_recogface_finger_yolo/Send positions to robot and unity/c calculation/Round 1 ==
  In1 : Inport
  Constant : Constant  Value=10000
  Divide : Product  Inputs=*/
  Multiply2 : Gain  Gain=10000
  Round2 : Rounding  Operator=round
  Out1 : Outport
  wires:
  Round2/1 -> Divide/1
  Constant/1 -> Divide/2
  Multiply2/1 -> Round2/1
  Divide/1 -> Out1/1
  In1/1 -> Multiply2/1

== matlab function Detailed_Simulation_recogface_finger_yolo/Lock_Unlock_Code ==
  data: locked input; button input; y output; angle input
function y = fcn(locked, button, angle)
coder.extrinsic('set_param');
%disp('teest');

if angle < 0.01 %if Heckklappe is closed
    if button == 0
        %if Locked is not equal to 0 then we change it
        if locked ~= 0
%            set_param('Detailed_Simulation_v13_Normal_Geschwindigkeit/Locked','Value','0');%LOCK
            set_param('Detailed_Simulation_aas_zhongying_nodecode/Locked','Value','0');%LOCK
        end
        %disp('Locked');
    else
        if locked ~= -1
%            set_param('Detailed_Simulation_v13_Normal_Geschwindigkeit/Locked','Value','-1');%UNLOCK
            set_param('Detailed_Simulation_aas_zhongying_nodecode/Locked','Value','-1');%LOCK
            %disp('Unlocked');
        end
    end
end
y = button;
